simulink model "ipLink"  (Simulink 7.4)
settings: Solver=FixedStepDiscrete  StartTime=0.0  StopTime=inf  FixedStep=1  RelTol=1e-3
settings Model: Creator=tyler  LastModifiedBy=tyler
settings RTWCC: SystemTargetFile=nrt.tlc  GenCodeOnly=on  TemplateMakefile=nrt_unix.tmf  Description=Nokia Real-Time Target  ProcessScript=nrt_make_rtw_hook
settings STFCustomTargetCC: ModelReferenceCompliant=off  GeneratePreprocessorConditionals=Disable all  MatFileLogging=on  SystemTargetFile=nrt.tlc
settings GRTTargetCC: ModelReferenceCompliant=off  ParMdlRefBuildCompliant=off  CompOptLevelCompliant=off
settings CustomProperty: DataType=string  Value=-lm -ldl
settings EnumStrPairs: String=PC

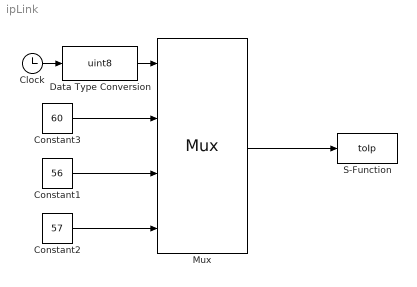
== system ipLink ==
  Clock : Clock
      settings: Decimation=10
  Constant1 : Constant  Value=56  OutDataTypeMode=uint8  OutDataType=fixdt(1, 16)  OutScaling=2^0  OutDataTypeStr=uint8
  Constant2 : Constant  Value=57  OutDataTypeMode=uint8  OutDataType=fixdt(1, 16)  OutScaling=2^0  OutDataTypeStr=uint8
  Constant3 : Constant  Value=60  OutDataTypeMode=uint8  OutDataType=fixdt(1, 16)  OutScaling=2^0  OutDataTypeStr=uint8
  Data Type Conversion : DataTypeConversion  OutDataTypeMode=uint8  OutDataType=fixdt(1, 16)  OutScaling=2^0  OutDataTypeStr=uint8
  Mux : Mux
  S-Function : S-Function  FunctionName=toIp  Parameters='153.104.47.61','6667'  EnableBusSupport=off
  wires:
  Constant1/1 -> Mux/3
  Constant2/1 -> Mux/4
  Constant3/1 -> Mux/2
  Clock/1 -> Data Type Conversion/1
  Data Type Conversion/1 -> Mux/1
  Mux/1 -> S-Function/1
